simulink subsystem "PieroControladoV"  (R2023b)
settings: Solver=VariableStepAuto  StartTime=0.0  StopTime=10.0  RelTol=1e-3
settings Model: Creator=Felix  LastModifiedBy=Daniel

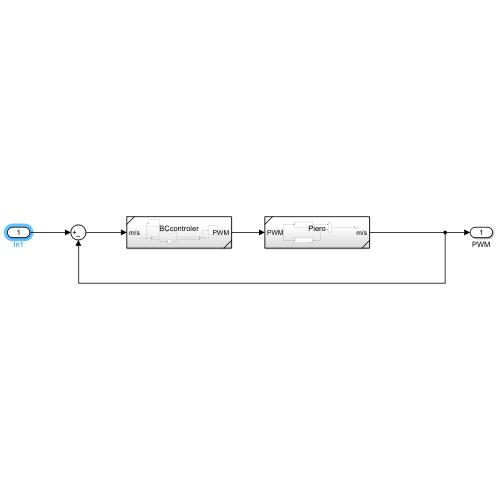
[thumbnail: Simulink's stored preview of the top-level diagram]
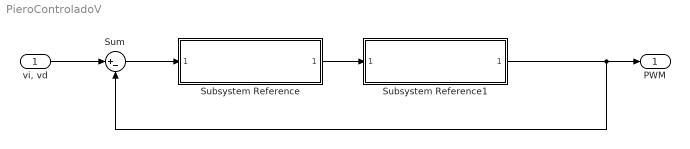
== system PieroControladoV ==
  "vi, vd" : Inport
  Subsystem Reference : Subsystem  ReferencedSubsystem=BCcontroler
  Subsystem Reference1 : Subsystem  ReferencedSubsystem=Piero
  Sum : Sum  Inputs=|+-
  PWM : Outport
  wires:
  "vi, vd"/1 -> Sum/1
  Sum/1 -> Subsystem Reference/1
  Subsystem Reference/1 -> Subsystem Reference1/1
  Subsystem Reference1/1 -> Sum/2, PWM/1
